simulink model "Problem_9"  (R2020a)
settings: Solver=VariableStepAuto  StartTime=0.0  StopTime=3  RelTol=1e-3
libraries: simulink x1
settings Model: Creator=Ganesh  LastModifiedBy=Ganesh

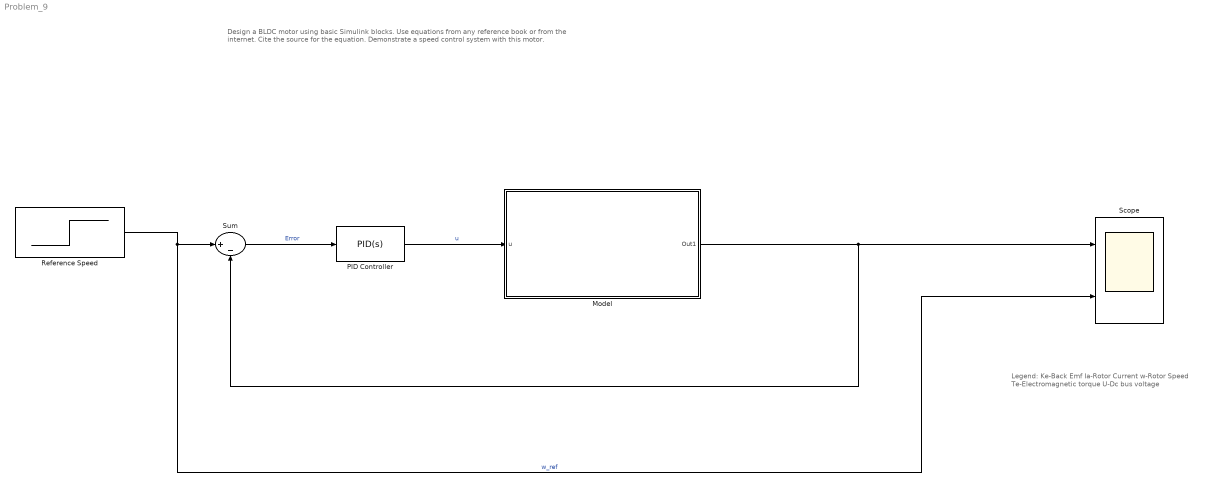
== system Problem_9 ==
  note: Legend:
      | Ke-Back Emf
      | Ia-Rotor Current
      | w-Rotor Speed
      | Te-Electromagnetic torque
      | U-Dc bus voltage
  note: Design a BLDC motor using basic Simulink blocks. Use equations from any reference book or from the internet. Cite the source for the equation. Demonstrate a speed control system with this motor.
  Model : Subsystem
  PID Controller : simulink/Continuous/PID Controller  Controller=PID  Form=Parallel  TimeDomain=Continuous-time  UseExternalTs=off  SampleTime=-1  IntegratorMethod=Forward Euler  FilterMethod=Forward Euler  ControllerParametersSource=internal  P=0.258758048387108  I=19.2352675000681  D=0.00057623058947149  UseFilter=on  N=9594.01098225587  TunerSelectOption=Transfer Function Based (PID Tuner App)  InitialConditionSource=internal  InitialConditionForIntegrator=0  InitialConditionForFilter=0  DifferentiatorICPrevScaledInput=0  ExternalReset=none  TrackingMode=off  Kt=1  LimitOutput=off  UpperSaturationLimit=inf  LowerSaturationLimit=-inf  LinearizeAsGain=on  AntiWindupMode=none  Kb=1  POutMin=[]  POutMax=[]  IOutMin=[]  IOutMax=[]  DOutMin=[]  DOutMax=[]  NOutMin=[]  NOutMax=[]  SumOutMin=[]  SumOutMax=[]  SaturationOutMin=[]  SaturationOutMax=[]  PParamMin=[]  PParamMax=[]  IParamMin=[]  IParamMax=[]  DParamMin=[]  DParamMax=[]  NParamMin=[]  NParamMax=[]  KbParamMin=[]  KbParamMax=[]  KtParamMin=[]  KtParamMax=[]  KbOutMin=[]  KbOutMax=[]  KtOutMin=[]  KtOutMax=[]  IntegratorOutMin=[]  IntegratorOutMax=[]  FilterOutMin=[]  FilterOutMax=[]  SumI1OutMin=[]  SumI1OutMax=[]  SumI2OutMin=[]  SumI2OutMax=[]  SumI3OutMin=[]  SumI3OutMax=[]  SumI4OutMin=[]  SumI4OutMax=[]  SumDOutMin=[]  SumDOutMax=[]  DifferentiatorOutMin=[]  DifferentiatorOutMax=[]  FilterDiffOutCoefMin=[]  FilterDiffOutCoefMax=[]  ReciprocalOutMin=[]  ReciprocalOutMax=[]  SumDenOutMin=[]  SumDenOutMax=[]  SumNumOutMin=[]  SumNumOutMax=[]  DivideOutMin=[]  DivideOutMax=[]  UdiffTsProdOutMin=[]  UdiffTsProdOutMax=[]  NTsProdOutMin=[]  NTsProdOutMax=[]  UintegralTsProdOutMin=[]  UintegralTsProdOutMax=[]  UngainTsProdOutMin=[]  UngainTsProdOutMax=[]  IntegratorContinuousStateAttributes=''  IntegratorStateMustResolveToSignalObject=off  IntegratorRTWStateStorageClass=Auto  FilterContinuousStateAttributes=''  FilterStateMustResolveToSignalObject=off  FilterRTWStateStorageClass=Auto  ParallelPVariant=InternalParameters  IdealPVariant=Disabled  IVariant=InternalParameters  DVariant=InternalParameters  IntegratorVariant=Continuous  SatVariant=Disabled  AWVariant=Passthrough  PCopyVariant=Disabled  TRVariant=Disabled  FdbkBlocksVariant=Forward  IdealPFdbkVariant=Disabled  SatFdbkVariant=Disabled  DerivativeFilterVariant=ContFilter  NVariant=InternalParameters  NCopyVariant=Disabled  FilterICVariant=InternalICsFilter  IntegratorICVariant=InternalICs  ExternalResetVariant=Disabled  TRSumVariant=Passthrough  SumFdbkVariant=Disabled  SumVariant=Sum_PID  TsampFilterVariant=InternalTs  TsampNgainVariant=Passthrough  TsampIntegralVariant=Passthrough
  Reference Speed : Step  After=1500  SampleTime=0
  Scope : Scope  NumInputPorts=2
  Sum : Sum  Inputs=|+-
  wires:
  Reference Speed/1 -> Scope/2, Sum/1  "w_ref"
  Sum/1 -> PID Controller/1  "Error"
  Model/1(Out1) -> Sum/2, Scope/1
  PID Controller/1 -> Model/1(u)  "u"

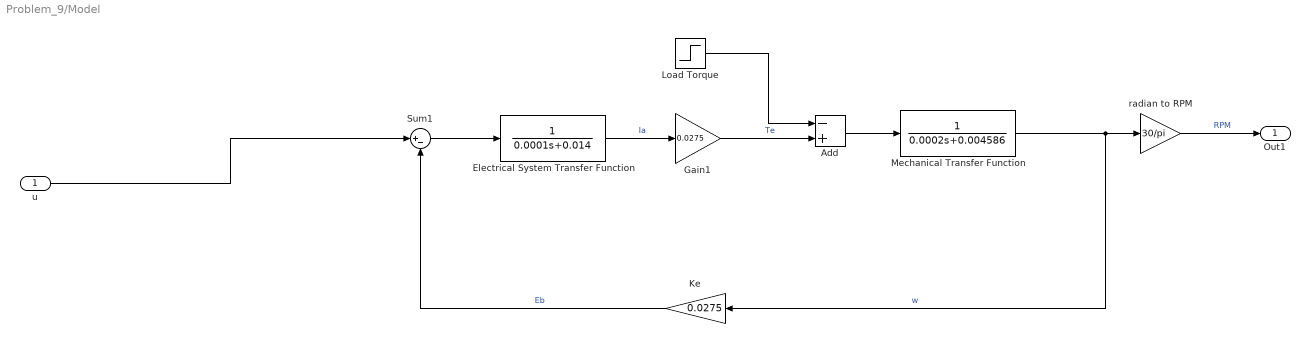
== system Problem_9/Model ==
  u : Inport
  Add : Sum  Inputs=-+
  Electrical System Transfer Function : TransferFcn  Denominator=[0.0001 0.014]
  Gain1 : Gain  Gain=0.0275
  Ke : Gain  Gain=0.0275
  Load Torque : Step  After=10  SampleTime=0
  Mechanical Transfer Function : TransferFcn  Denominator=[0.0002 0.004586]
  Sum1 : Sum  Inputs=|+-
  radian to RPM : Gain  Gain=30/pi
  Out1 : Outport
  wires:
  Electrical System Transfer Function/1 -> Gain1/1  "Ia"
  Load Torque/1 -> Add/1
  Ke/1 -> Sum1/2  "Eb"
  u/1 -> Sum1/1
  Add/1 -> Mechanical Transfer Function/1
  Mechanical Transfer Function/1 -> Ke/1, radian to RPM/1  "w"
  Gain1/1 -> Add/2  "Te"
  Sum1/1 -> Electrical System Transfer Function/1
  radian to RPM/1 -> Out1/1  "RPM"
